simulink model "model1"  (R2024b)
settings: Solver=VariableStepAuto  StartTime=0.0  StopTime=10.0  MaxStep=1e-3  RelTol=1e-3
settings Model: Creator=mehmetcanevi  LastModifiedBy=mehmetcanevi

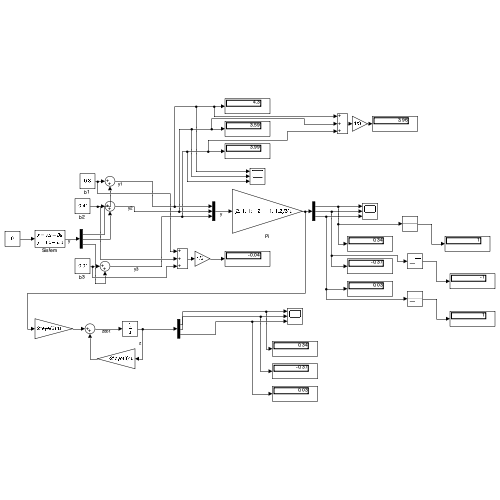
[thumbnail: Simulink's stored preview of the top-level diagram]
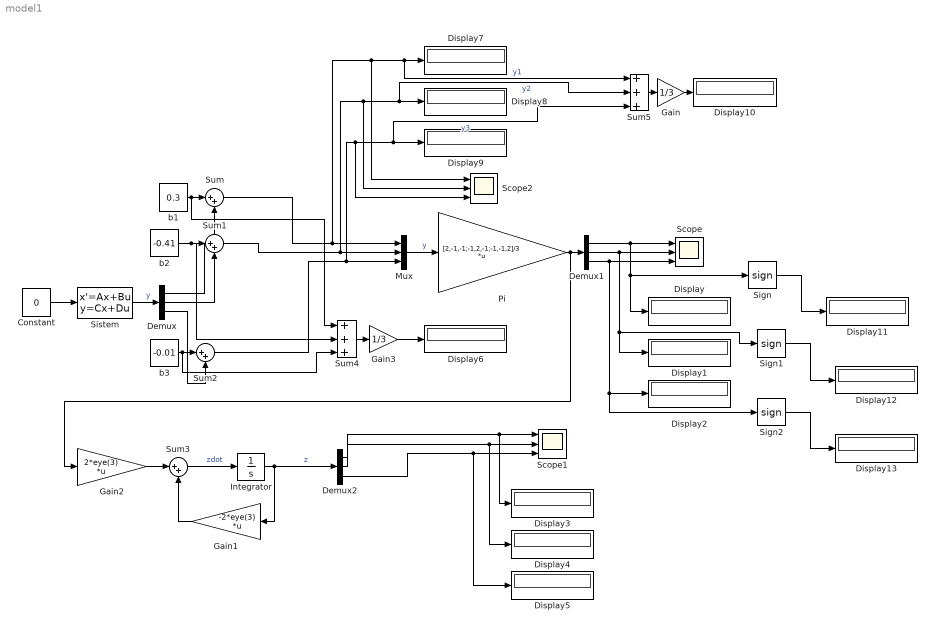
== system model1 ==
  Constant : Constant  Value=0
  Demux : Demux  Outputs=3
  Demux1 : Demux  Outputs=3
  Demux2 : Demux  Outputs=3
  Display{,1..13} (14 alike) : Display
  Gain : Gain  Gain=1/3
  Gain1 : Gain  Gain=-2*eye(3)  Multiplication=Matrix(K*u)
  Gain2 : Gain  Gain=2*eye(3)  Multiplication=Matrix(K*u)
  Gain3 : Gain  Gain=1/3
  Integrator : Integrator
  Mux : Mux  Inputs=3
  Pi : Gain  Gain=[2,-1,-1;-1,2,-1;-1,-1,2]/3  Multiplication=Matrix(K*u)
  Scope : Scope  NumInputPorts=3
  Scope1 : Scope  NumInputPorts=3
  Scope2 : Scope  NumInputPorts=3
  Sign : Signum
  Sign1 : Signum
  Sign2 : Signum
  Sistem : StateSpace  A=0  B=0  C=[1;1;1]  D=[0;0;0]  InitialCondition=4
  Sum{,1..3} (4 alike) : Sum  Inputs=|++
  Sum4 : Sum  Inputs=+++
  Sum5 : Sum  Inputs=+++
  b1 : Constant  Value=0.3
  b2 : Constant  Value=-0.41
  b3 : Constant  Value=-0.01
  wires:
  Constant/1 -> Sistem/1
  Sistem/1 -> Demux/1  "y"
  b1/1 -> Sum4/1, Sum/1
  Demux/1 -> Sum/2
  b2/1 -> Sum4/2, Sum1/1
  Demux/2 -> Sum1/2
  b3/1 -> Sum4/3, Sum2/1
  Demux/3 -> Sum2/2
  Sum2/1 -> Scope2/3, Sum5/3, Display9/1, Mux/3  "y3"
  Sum1/1 -> Scope2/2, Sum5/2, Display8/1, Mux/2  "y2"
  Sum/1 -> Scope2/1, Sum5/1, Display7/1, Mux/1  "y1"
  Mux/1 -> Pi/1  "y"
  Pi/1 -> Gain2/1, Demux1/1
  Demux1/1 -> Sign/1, Display/1, Scope/1
  Demux1/2 -> Sign1/1, Display1/1, Scope/2
  Demux1/3 -> Sign2/1, Display2/1, Scope/3
  Sum3/1 -> Integrator/1  "zdot"
  Integrator/1 -> Demux2/1, Gain1/1  "z"
  Gain1/1 -> Sum3/2
  Demux2/1 -> Display3/1, Scope1/1
  Demux2/2 -> Display4/1, Scope1/2
  Demux2/3 -> Display5/1, Scope1/3
  Gain2/1 -> Sum3/1
  Sum5/1 -> Gain/1
  Gain/1 -> Display10/1
  Sum4/1 -> Gain3/1
  Gain3/1 -> Display6/1
  Sign/1 -> Display11/1
  Sign1/1 -> Display12/1
  Sign2/1 -> Display13/1
